simulink subsystem "transmitter"  (R2021b)
settings: Solver=VariableStepAuto  StartTime=0.0  StopTime=10.0  RelTol=1e-3
settings Model: Creator=torha  LastModifiedBy=torha

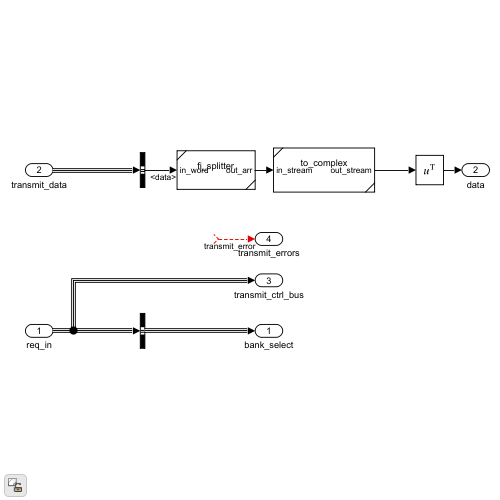
[thumbnail: Simulink's stored preview of the top-level diagram]
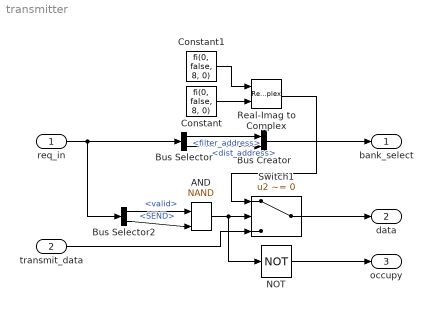
== system transmitter ==
  req_in : Inport
  transmit_data : Inport  Port=2
  AND : Logic  Operator=NAND  IconShape=distinctive  AllPortsSameDT=off  OutDataTypeStr=boolean
  Bus Creator : BusCreator  Inputs=2
  Bus Selector : BusSelector  OutputSignals=filter_address,dist_address
  Bus Selector2 : BusSelector  OutputSignals=valid,SEND
  Constant : Constant  Value=fi(0, false, 8, 0)
  Constant1 : Constant  Value=fi(0, false, 8, 0)
  NOT : Logic  Operator=NOT  IconShape=distinctive  AllPortsSameDT=off  OutDataTypeStr=boolean
  Real-Imag to Complex : RealImagToComplex
  Switch1 : Switch  Criteria=u2 ~= 0
  bank_select : Outport
  data : Outport  Port=2
  occupy : Outport  Port=3
  wires:
  Constant/1 -> Real-Imag to Complex/2
  Constant1/1 -> Real-Imag to Complex/1
  NOT/1 -> occupy/1
  AND/1 -> NOT/1, Switch1/2
  Real-Imag to Complex/1 -> Switch1/1
  Bus Selector2/2 -> AND/2  "<SEND>"
  Bus Selector2/1 -> AND/1  "<valid>"
  req_in/1 -> Bus Selector/1, Bus Selector2/1
  Bus Creator/1 -> bank_select/1
  transmit_data/1 -> Switch1/3
  Switch1/1 -> data/1
  Bus Selector/1 -> Bus Creator/1  "<filter_address>"
  Bus Selector/2 -> Bus Creator/2  "<dist_address>"
